simulink model "TST_Brk_DD"  (R2016b)
settings: Solver=FixedStepDiscrete  StartTime=0.0  StopTime=simTime  FixedStep=sampleTime  RelTol=1e-3
values from neighbouring files (symbols this model uses):
  testCase = 1    [initTST_Brk_DD_001.m]    (also in initTST_Brk_DD_002.m = 2; initTST_Brk_DD_003.m = 3)
libraries: simulink x4
settings Model: Creator=wolf072601  LastModifiedBy=wolf072601
settings DebuggingCC: SignalRangeChecking=error

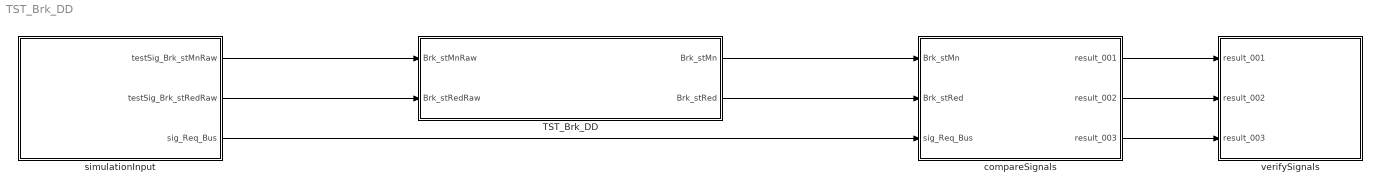
== system TST_Brk_DD ==
  TST_Brk_DD : Subsystem
  compareSignals : Subsystem
  simulationInput : Subsystem
  verifySignals : Subsystem
  wires:
  simulationInput/1(testSig_Brk_stMnRaw) -> TST_Brk_DD/1(Brk_stMnRaw)
  simulationInput/2(testSig_Brk_stRedRaw) -> TST_Brk_DD/2(Brk_stRedRaw)
  TST_Brk_DD/1(Brk_stMn) -> compareSignals/1(Brk_stMn)
  TST_Brk_DD/2(Brk_stRed) -> compareSignals/2(Brk_stRed)
  simulationInput/3(sig_Req_Bus) -> compareSignals/3(sig_Req_Bus)
  compareSignals/1(result_001) -> verifySignals/1(result_001)
  compareSignals/2(result_002) -> verifySignals/2(result_002)
  compareSignals/3(result_003) -> verifySignals/3(result_003)

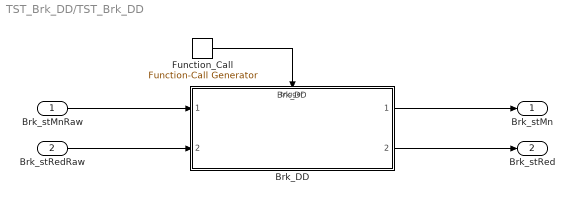
== system TST_Brk_DD/TST_Brk_DD ==
  Brk_stMnRaw : Inport
  Brk_stRedRaw : Inport  Port=2
  Brk_DD : ModelReference  ModelNameDialog=Brk_DD  ModelReferenceVersion=1.5  TriggerPortName=function  TriggerPortTriggerType=function-call  TriggerPortStatesWhenEnabling=held
  Function_Call : simulink/Ports & Subsystems/Function-Call Generator  sample_time=sampleTime  numberOfIterations=1
  Brk_stMn : Outport
  Brk_stRed : Outport  Port=2
  wires:
  Function_Call/1 -> Brk_DD/Trigger
  Brk_stMnRaw/1 -> Brk_DD/1
  Brk_stRedRaw/1 -> Brk_DD/2
  Brk_DD/1 -> Brk_stMn/1
  Brk_DD/2 -> Brk_stRed/1

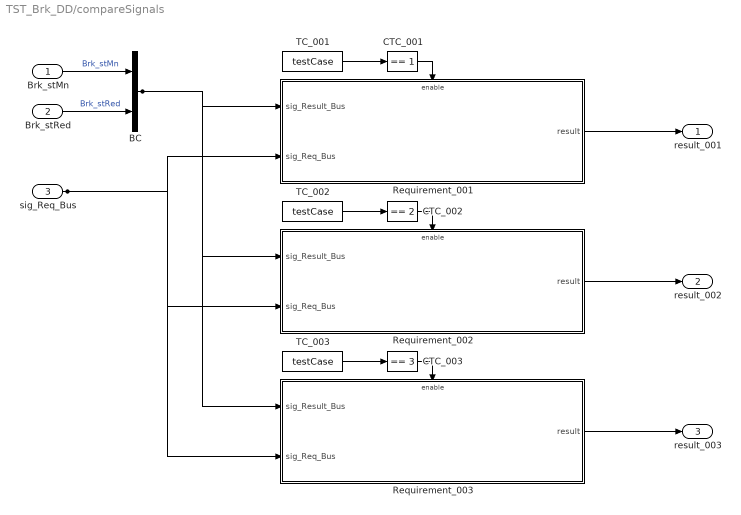
== system TST_Brk_DD/compareSignals ==
  Brk_stMn : Inport
  Brk_stRed : Inport  Port=2
  sig_Req_Bus : Inport  Port=3
  BC : BusCreator  Inputs=2
  CTC_001 : simulink/Logic and Bit Operations/Compare To Constant  relop===  const=1  OutDataTypeStr=boolean
  CTC_002 : simulink/Logic and Bit Operations/Compare To Constant  relop===  const=2  OutDataTypeStr=boolean
  CTC_003 : simulink/Logic and Bit Operations/Compare To Constant  relop===  const=3  OutDataTypeStr=boolean
  Requirement_001 : Subsystem
  Requirement_002 : Subsystem
  Requirement_003 : Subsystem
  TC_001 : Constant  Value=testCase
  TC_002 : Constant  Value=testCase
  TC_003 : Constant  Value=testCase
  result_001 : Outport
  result_002 : Outport  Port=2
  result_003 : Outport  Port=3
  wires:
  Brk_stMn/1 -> BC/1  "Brk_stMn"
  Brk_stRed/1 -> BC/2  "Brk_stRed"
  TC_001/1 -> CTC_001/1
  CTC_001/1 -> Requirement_001/Enable
  sig_Req_Bus/1 -> Requirement_001/2(sig_Req_Bus), Requirement_002/2(sig_Req_Bus), Requirement_003/2(sig_Req_Bus)
  BC/1 -> Requirement_001/1(sig_Result_Bus), Requirement_002/1(sig_Result_Bus), Requirement_003/1(sig_Result_Bus)
  Requirement_001/1(result) -> result_001/1
  TC_002/1 -> CTC_002/1
  CTC_002/1 -> Requirement_002/Enable
  Requirement_002/1(result) -> result_002/1
  TC_003/1 -> CTC_003/1
  CTC_003/1 -> Requirement_003/Enable
  Requirement_003/1(result) -> result_003/1

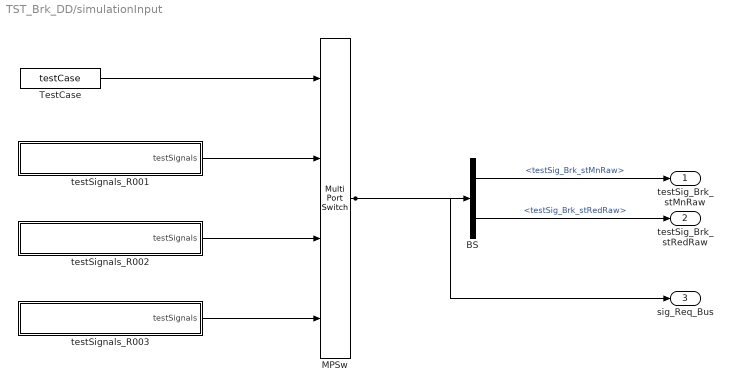
== system TST_Brk_DD/simulationInput ==
  BS : BusSelector  OutputSignals=testSig_Brk_stMnRaw,testSig_Brk_stRedRaw
  MPSw : MultiPortSwitch  SaturateOnIntegerOverflow=on  InputSameDT=on
  TestCase : Constant  Value=testCase
  testSignals_R001 : Subsystem
  testSignals_R002 : Subsystem
  testSignals_R003 : Subsystem
  testSig_Brk_stMnRaw : Outport
  testSig_Brk_stRedRaw : Outport  Port=2
  sig_Req_Bus : Outport  Port=3
  wires:
  BS/1 -> testSig_Brk_stMnRaw/1  "<testSig_Brk_stMnRaw>"
  BS/2 -> testSig_Brk_stRedRaw/1  "<testSig_Brk_stRedRaw>"
  MPSw/1 -> BS/1, sig_Req_Bus/1
  TestCase/1 -> MPSw/1
  testSignals_R001/1(testSignals) -> MPSw/2
  testSignals_R002/1(testSignals) -> MPSw/3
  testSignals_R003/1(testSignals) -> MPSw/4

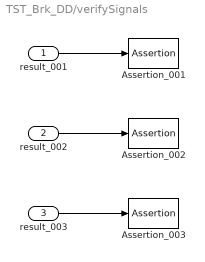
== system TST_Brk_DD/verifySignals ==
  result_001 : Inport
  result_002 : Inport  Port=2
  result_003 : Inport  Port=3
  Assertion_001 : Assertion  Enabled=off
  Assertion_002 : Assertion  Enabled=off
  Assertion_003 : Assertion  Enabled=off
  wires:
  result_001/1 -> Assertion_001/1
  result_002/1 -> Assertion_002/1
  result_003/1 -> Assertion_003/1

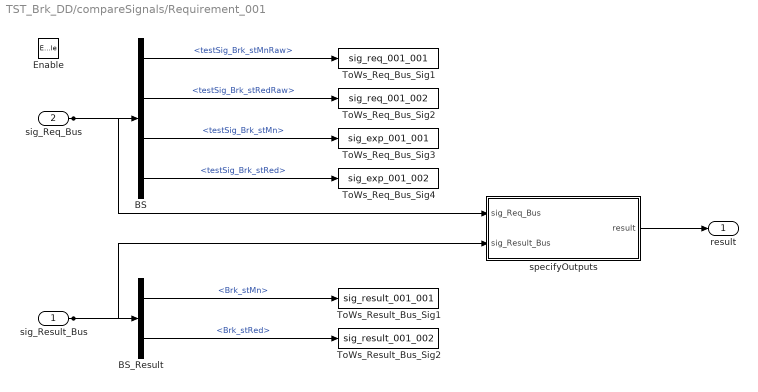
== system TST_Brk_DD/compareSignals/Requirement_001 ==
  sig_Result_Bus : Inport
  sig_Req_Bus : Inport  Port=2
  Enable : EnablePort
  BS : BusSelector  OutputSignals=testSig_Brk_stMnRaw,testSig_Brk_stRedRaw,testSig_Brk_stMn,testSig_Brk_stRed
  BS_Result : BusSelector  OutputSignals=Brk_stMn,Brk_stRed
  ToWs_Req_Bus_Sig1 : ToWorkspace  VariableName=sig_req_001_001  SaveFormat=Structure With Time
  ToWs_Req_Bus_Sig2 : ToWorkspace  VariableName=sig_req_001_002  SaveFormat=Structure With Time
  ToWs_Req_Bus_Sig3 : ToWorkspace  VariableName=sig_exp_001_001  SaveFormat=Structure With Time
  ToWs_Req_Bus_Sig4 : ToWorkspace  VariableName=sig_exp_001_002  SaveFormat=Structure With Time
  ToWs_Result_Bus_Sig1 : ToWorkspace  VariableName=sig_result_001_001  SaveFormat=Structure With Time
  ToWs_Result_Bus_Sig2 : ToWorkspace  VariableName=sig_result_001_002  SaveFormat=Structure With Time
  specifyOutputs : Subsystem
  result : Outport
  wires:
  sig_Req_Bus/1 -> BS/1, specifyOutputs/1(sig_Req_Bus)
  BS/1 -> ToWs_Req_Bus_Sig1/1  "<testSig_Brk_stMnRaw>"
  BS/2 -> ToWs_Req_Bus_Sig2/1  "<testSig_Brk_stRedRaw>"
  BS/3 -> ToWs_Req_Bus_Sig3/1  "<testSig_Brk_stMn>"
  BS/4 -> ToWs_Req_Bus_Sig4/1  "<testSig_Brk_stRed>"
  sig_Result_Bus/1 -> BS_Result/1, specifyOutputs/2(sig_Result_Bus)
  BS_Result/1 -> ToWs_Result_Bus_Sig1/1  "<Brk_stMn>"
  BS_Result/2 -> ToWs_Result_Bus_Sig2/1  "<Brk_stRed>"
  specifyOutputs/1(result) -> result/1

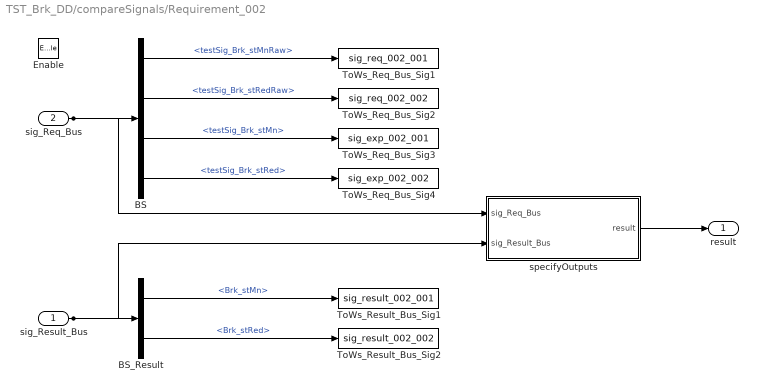
== system TST_Brk_DD/compareSignals/Requirement_002 ==
  sig_Result_Bus : Inport
  sig_Req_Bus : Inport  Port=2
  Enable : EnablePort
  BS : BusSelector  OutputSignals=testSig_Brk_stMnRaw,testSig_Brk_stRedRaw,testSig_Brk_stMn,testSig_Brk_stRed
  BS_Result : BusSelector  OutputSignals=Brk_stMn,Brk_stRed
  ToWs_Req_Bus_Sig1 : ToWorkspace  VariableName=sig_req_002_001  SaveFormat=Structure With Time
  ToWs_Req_Bus_Sig2 : ToWorkspace  VariableName=sig_req_002_002  SaveFormat=Structure With Time
  ToWs_Req_Bus_Sig3 : ToWorkspace  VariableName=sig_exp_002_001  SaveFormat=Structure With Time
  ToWs_Req_Bus_Sig4 : ToWorkspace  VariableName=sig_exp_002_002  SaveFormat=Structure With Time
  ToWs_Result_Bus_Sig1 : ToWorkspace  VariableName=sig_result_002_001  SaveFormat=Structure With Time
  ToWs_Result_Bus_Sig2 : ToWorkspace  VariableName=sig_result_002_002  SaveFormat=Structure With Time
  specifyOutputs : Subsystem
  result : Outport
  wires:
  sig_Req_Bus/1 -> BS/1, specifyOutputs/1(sig_Req_Bus)
  BS/1 -> ToWs_Req_Bus_Sig1/1  "<testSig_Brk_stMnRaw>"
  BS/2 -> ToWs_Req_Bus_Sig2/1  "<testSig_Brk_stRedRaw>"
  BS/3 -> ToWs_Req_Bus_Sig3/1  "<testSig_Brk_stMn>"
  BS/4 -> ToWs_Req_Bus_Sig4/1  "<testSig_Brk_stRed>"
  sig_Result_Bus/1 -> BS_Result/1, specifyOutputs/2(sig_Result_Bus)
  BS_Result/1 -> ToWs_Result_Bus_Sig1/1  "<Brk_stMn>"
  BS_Result/2 -> ToWs_Result_Bus_Sig2/1  "<Brk_stRed>"
  specifyOutputs/1(result) -> result/1

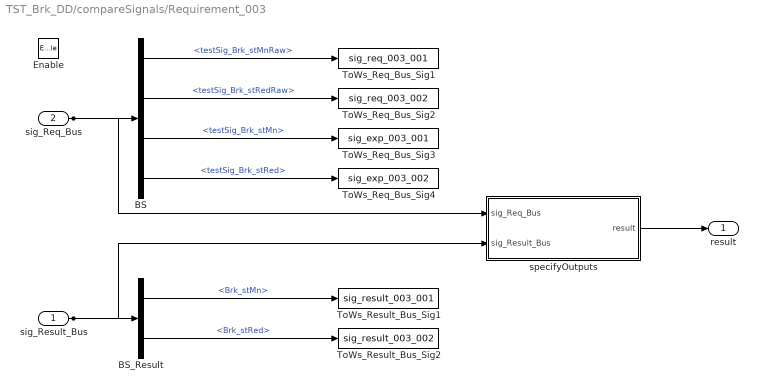
== system TST_Brk_DD/compareSignals/Requirement_003 ==
  sig_Result_Bus : Inport
  sig_Req_Bus : Inport  Port=2
  Enable : EnablePort
  BS : BusSelector  OutputSignals=testSig_Brk_stMnRaw,testSig_Brk_stRedRaw,testSig_Brk_stMn,testSig_Brk_stRed
  BS_Result : BusSelector  OutputSignals=Brk_stMn,Brk_stRed
  ToWs_Req_Bus_Sig1 : ToWorkspace  VariableName=sig_req_003_001  SaveFormat=Structure With Time
  ToWs_Req_Bus_Sig2 : ToWorkspace  VariableName=sig_req_003_002  SaveFormat=Structure With Time
  ToWs_Req_Bus_Sig3 : ToWorkspace  VariableName=sig_exp_003_001  SaveFormat=Structure With Time
  ToWs_Req_Bus_Sig4 : ToWorkspace  VariableName=sig_exp_003_002  SaveFormat=Structure With Time
  ToWs_Result_Bus_Sig1 : ToWorkspace  VariableName=sig_result_003_001  SaveFormat=Structure With Time
  ToWs_Result_Bus_Sig2 : ToWorkspace  VariableName=sig_result_003_002  SaveFormat=Structure With Time
  specifyOutputs : Subsystem
  result : Outport
  wires:
  sig_Req_Bus/1 -> BS/1, specifyOutputs/1(sig_Req_Bus)
  BS/1 -> ToWs_Req_Bus_Sig1/1  "<testSig_Brk_stMnRaw>"
  BS/2 -> ToWs_Req_Bus_Sig2/1  "<testSig_Brk_stRedRaw>"
  BS/3 -> ToWs_Req_Bus_Sig3/1  "<testSig_Brk_stMn>"
  BS/4 -> ToWs_Req_Bus_Sig4/1  "<testSig_Brk_stRed>"
  sig_Result_Bus/1 -> BS_Result/1, specifyOutputs/2(sig_Result_Bus)
  BS_Result/1 -> ToWs_Result_Bus_Sig1/1  "<Brk_stMn>"
  BS_Result/2 -> ToWs_Result_Bus_Sig2/1  "<Brk_stRed>"
  specifyOutputs/1(result) -> result/1

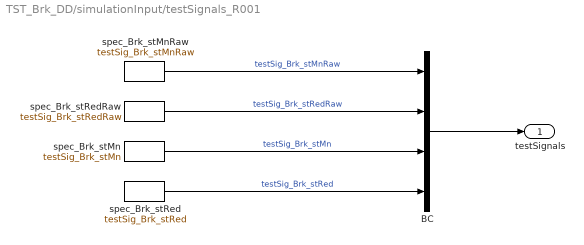
== system TST_Brk_DD/simulationInput/testSignals_R001 ==
  BC : BusCreator  Inputs=4
  spec_Brk_stMn : FromWorkspace  VariableName=testSig_Brk_stMn  Interpolate=off  OutputAfterFinalValue=Holding final value
  spec_Brk_stMnRaw : FromWorkspace  VariableName=testSig_Brk_stMnRaw  Interpolate=off  OutputAfterFinalValue=Holding final value
  spec_Brk_stRed : FromWorkspace  VariableName=testSig_Brk_stRed  Interpolate=off  OutputAfterFinalValue=Holding final value
  spec_Brk_stRedRaw : FromWorkspace  VariableName=testSig_Brk_stRedRaw  Interpolate=off  OutputAfterFinalValue=Holding final value
  testSignals : Outport
  wires:
  BC/1 -> testSignals/1
  spec_Brk_stMnRaw/1 -> BC/1  "testSig_Brk_stMnRaw"
  spec_Brk_stRedRaw/1 -> BC/2  "testSig_Brk_stRedRaw"
  spec_Brk_stMn/1 -> BC/3  "testSig_Brk_stMn"
  spec_Brk_stRed/1 -> BC/4  "testSig_Brk_stRed"

== system TST_Brk_DD/simulationInput/testSignals_R002 ==
  BC : BusCreator  Inputs=4
  spec_Brk_stMn : FromWorkspace  VariableName=testSig_Brk_stMn  Interpolate=off  OutputAfterFinalValue=Holding final value
  spec_Brk_stMnRaw : FromWorkspace  VariableName=testSig_Brk_stMnRaw  Interpolate=off  OutputAfterFinalValue=Holding final value
  spec_Brk_stRed : FromWorkspace  VariableName=testSig_Brk_stRed  Interpolate=off  OutputAfterFinalValue=Holding final value
  spec_Brk_stRedRaw : FromWorkspace  VariableName=testSig_Brk_stRedRaw  Interpolate=off  OutputAfterFinalValue=Holding final value
  testSignals : Outport
  wires:
  BC/1 -> testSignals/1
  spec_Brk_stMnRaw/1 -> BC/1  "testSig_Brk_stMnRaw"
  spec_Brk_stRedRaw/1 -> BC/2  "testSig_Brk_stRedRaw"
  spec_Brk_stMn/1 -> BC/3  "testSig_Brk_stMn"
  spec_Brk_stRed/1 -> BC/4  "testSig_Brk_stRed"

== system TST_Brk_DD/simulationInput/testSignals_R003 ==
  BC : BusCreator  Inputs=4
  spec_Brk_stMn : FromWorkspace  VariableName=testSig_Brk_stMn  Interpolate=off  OutputAfterFinalValue=Holding final value
  spec_Brk_stMnRaw : FromWorkspace  VariableName=testSig_Brk_stMnRaw  Interpolate=off  OutputAfterFinalValue=Holding final value
  spec_Brk_stRed : FromWorkspace  VariableName=testSig_Brk_stRed  Interpolate=off  OutputAfterFinalValue=Holding final value
  spec_Brk_stRedRaw : FromWorkspace  VariableName=testSig_Brk_stRedRaw  Interpolate=off  OutputAfterFinalValue=Holding final value
  testSignals : Outport
  wires:
  BC/1 -> testSignals/1
  spec_Brk_stMnRaw/1 -> BC/1  "testSig_Brk_stMnRaw"
  spec_Brk_stRedRaw/1 -> BC/2  "testSig_Brk_stRedRaw"
  spec_Brk_stMn/1 -> BC/3  "testSig_Brk_stMn"
  spec_Brk_stRed/1 -> BC/4  "testSig_Brk_stRed"

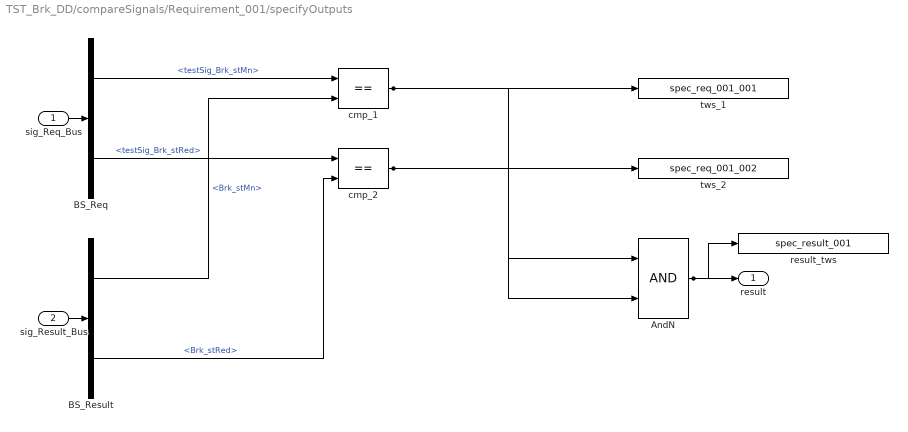
== system TST_Brk_DD/compareSignals/Requirement_001/specifyOutputs ==
  sig_Req_Bus : Inport
  sig_Result_Bus : Inport  Port=2
  AndN : Logic
  BS_Req : BusSelector  OutputSignals=testSig_Brk_stMn,testSig_Brk_stRed
  BS_Result : BusSelector  OutputSignals=Brk_stMn,Brk_stRed
  cmp_1 : RelationalOperator  Operator===  RndMeth=Nearest  InputSameDT=on
  cmp_2 : RelationalOperator  Operator===  RndMeth=Nearest  InputSameDT=on
  result_tws : ToWorkspace  VariableName=spec_result_001
  tws_1 : ToWorkspace  VariableName=spec_req_001_001
  tws_2 : ToWorkspace  VariableName=spec_req_001_002
  result : Outport
  wires:
  sig_Req_Bus/1 -> BS_Req/1
  sig_Result_Bus/1 -> BS_Result/1
  AndN/1 -> result/1, result_tws/1
  BS_Req/1 -> cmp_1/1  "<testSig_Brk_stMn>"
  BS_Result/1 -> cmp_1/2  "<Brk_stMn>"
  cmp_1/1 -> tws_1/1, AndN/1
  BS_Req/2 -> cmp_2/1  "<testSig_Brk_stRed>"
  BS_Result/2 -> cmp_2/2  "<Brk_stRed>"
  cmp_2/1 -> tws_2/1, AndN/2

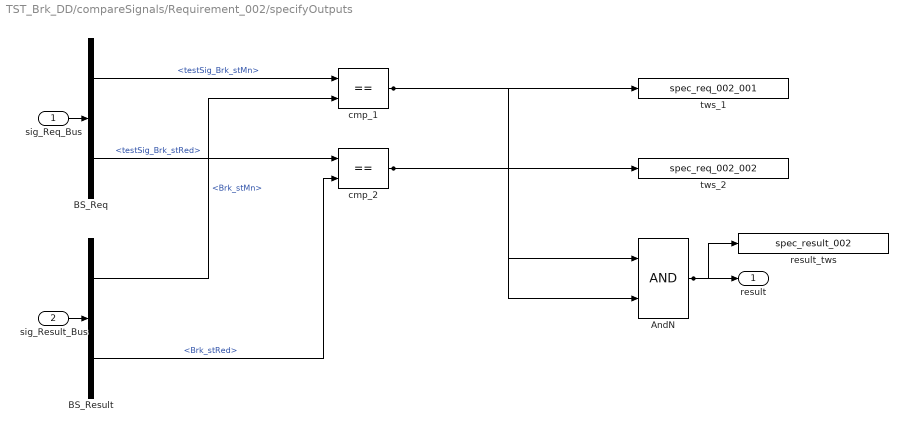
== system TST_Brk_DD/compareSignals/Requirement_002/specifyOutputs ==
  sig_Req_Bus : Inport
  sig_Result_Bus : Inport  Port=2
  AndN : Logic
  BS_Req : BusSelector  OutputSignals=testSig_Brk_stMn,testSig_Brk_stRed
  BS_Result : BusSelector  OutputSignals=Brk_stMn,Brk_stRed
  cmp_1 : RelationalOperator  Operator===  RndMeth=Nearest  InputSameDT=on
  cmp_2 : RelationalOperator  Operator===  RndMeth=Nearest  InputSameDT=on
  result_tws : ToWorkspace  VariableName=spec_result_002
  tws_1 : ToWorkspace  VariableName=spec_req_002_001
  tws_2 : ToWorkspace  VariableName=spec_req_002_002
  result : Outport
  wires:
  sig_Req_Bus/1 -> BS_Req/1
  sig_Result_Bus/1 -> BS_Result/1
  AndN/1 -> result/1, result_tws/1
  BS_Req/1 -> cmp_1/1  "<testSig_Brk_stMn>"
  BS_Result/1 -> cmp_1/2  "<Brk_stMn>"
  cmp_1/1 -> tws_1/1, AndN/1
  BS_Req/2 -> cmp_2/1  "<testSig_Brk_stRed>"
  BS_Result/2 -> cmp_2/2  "<Brk_stRed>"
  cmp_2/1 -> tws_2/1, AndN/2

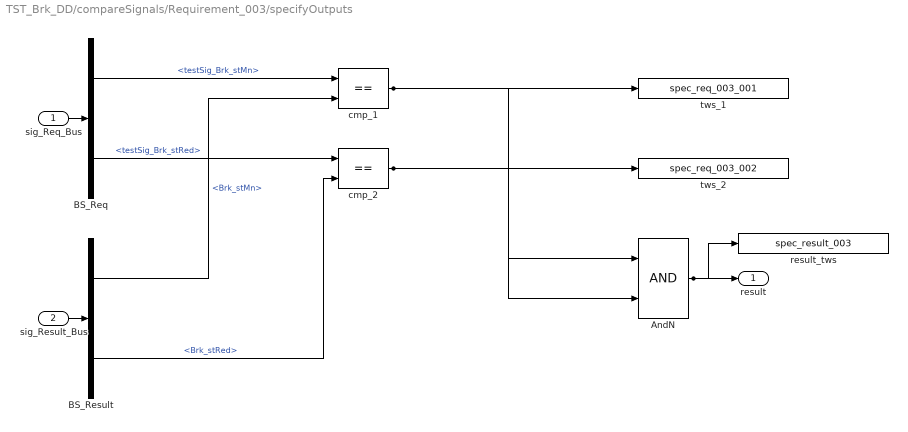
== system TST_Brk_DD/compareSignals/Requirement_003/specifyOutputs ==
  sig_Req_Bus : Inport
  sig_Result_Bus : Inport  Port=2
  AndN : Logic
  BS_Req : BusSelector  OutputSignals=testSig_Brk_stMn,testSig_Brk_stRed
  BS_Result : BusSelector  OutputSignals=Brk_stMn,Brk_stRed
  cmp_1 : RelationalOperator  Operator===  RndMeth=Nearest  InputSameDT=on
  cmp_2 : RelationalOperator  Operator===  RndMeth=Nearest  InputSameDT=on
  result_tws : ToWorkspace  VariableName=spec_result_003
  tws_1 : ToWorkspace  VariableName=spec_req_003_001
  tws_2 : ToWorkspace  VariableName=spec_req_003_002
  result : Outport
  wires:
  sig_Req_Bus/1 -> BS_Req/1
  sig_Result_Bus/1 -> BS_Result/1
  AndN/1 -> result/1, result_tws/1
  BS_Req/1 -> cmp_1/1  "<testSig_Brk_stMn>"
  BS_Result/1 -> cmp_1/2  "<Brk_stMn>"
  cmp_1/1 -> tws_1/1, AndN/1
  BS_Req/2 -> cmp_2/1  "<testSig_Brk_stRed>"
  BS_Result/2 -> cmp_2/2  "<Brk_stRed>"
  cmp_2/1 -> tws_2/1, AndN/2
